simulink model "NMPC_4VEH_4TL"  (R2022b)
settings: Solver=ode4  StartTime=0.0  StopTime=1950  FixedStep=0.1  RelTol=1e-3
PostLoadFcn:
  | , if any(exist('dsrtsu_mdlpostloadfcn', 'file') == [2, 3, 6]), try dsrtsu_mdlpostloadfcn('Execute', bdroot); catch fprintf('Error in PostLoadFcn (dsrtsu_mdlpostloadfcn) for model "%s":\n %s\n', bdroot, lasterr); end, end,
values from neighbouring files (symbols this model uses):
  k_road_map = k_road_map(:)    [NMPC_init_4veh_4TL.m]
  N = 35    [ACADO_4veh_4TL.m]    (also in ACADO_4veh_4TL_BACKUP.m; NMPC_chebyshev_grid.m; NMPC_init_4veh_4TL.m; debug_vincoli_violati.m = 40)
  N_iter = 1    [NMPC_init_4veh_4TL.m]
  N_Jterms = length(Qx1)    [NMPC_init_4veh_4TL.m]
  NMPC_Wmat1 = reshape(W1.',1,[])    [NMPC_init_4veh_4TL.m]
  NMPC_WNmat1 = reshape(WN1.',1,[])    [NMPC_init_4veh_4TL.m]
  t_dwell = 7    [ACADO_4veh_4TL.m]    (also in ACADO_4veh_4TL_BACKUP.m; NMPC_init_4veh_4TL.m)
  t_offset = 0    [NMPC_init_4veh_4TL.m]
  time_bag_sim = (0:1:round(time_bag(end))-1)'    [NMPC_init_4veh_4TL.m]
  time_grid = T_hor*tau_grid    [NMPC_init_4veh_4TL.m]
  tl_state_sim = zeros(round(time_bag(end))-1,size(tl_col,2))    [NMPC_init_4veh_4TL.m]
  Ts = Ts_ctrl    (= 1)    [NMPC_init_4veh_4TL.m]
  Vmax = 50    [NMPC_init_4veh_4TL.m]
  xInit = [0 0 0 -9 0 0 -19 0 0 -29 0 0]    [NMPC_init_4veh_4TL.m]
undefined symbols (not defined in the file or in its folder): ds, s_start
libraries: simulink x1
(part 1 of 2)
settings Model: DSRTSU_INTERNAL_RTI_VER=450  DSRTSU_INTERNAL_RTI_TYPE=rti1401  DSRTSU_INTERNAL_RTIFPGA=40  Creator=d068515  LastModifiedBy=ricca
settings DataIOCC: SaveFormat=StructureWithTime
settings OptimizationCC: BlockReduction=off  LifeSpan=inf
settings DebuggingCC: SFExecutionAtInitializationDiag=none  SFMachineParentedDataDiag=warning  ArithmeticOperatorsInVariantConditions=warning
settings HardwareCC: ProdBitPerSizeT=32  ProdBitPerPtrDiffT=32  ProdEndianess=BigEndian  ProdWordSize=32  ProdHWDeviceType=Generic->Custom  TargetIntDivRoundTo=Zero  TargetEndianess=BigEndian  TargetHWDeviceType=Generic->Custom
settings SFSimCC: CustomCodeUndefinedFunction=UseInterfaceOnly
settings RTWCC: Description=dSPACE DS1401 Hardware Platform  SystemTargetFile=rti1401.tlc  MakeCommand=make_rti  TemplateMakefile=rti1401.tmf
settings CodeAppCC: StateflowObjectComments=on
settings STFCustomTargetCC: ParMdlRefBuildCompliant=on  GRTInterface=on  SystemTargetFile=rti1401.tlc
settings GRTTargetCC: TargetLangStandard=C89/C90 (ANSI)  CompOptLevelCompliant=off  ConcurrentExecutionCompliant=off  CombineOutputUpdateFcns=off  MatFileLogging=off  CPPClassGenCompliant=off  GRTInterface=on  UseToolchainInfoCompliant=off  ExtModeMexFile=noextcomm

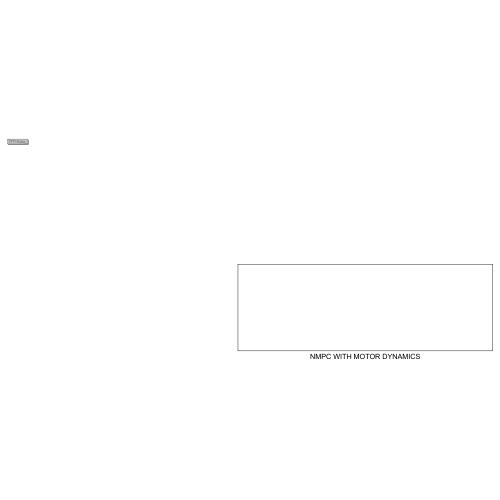
[thumbnail: Simulink's stored preview of the top-level diagram]
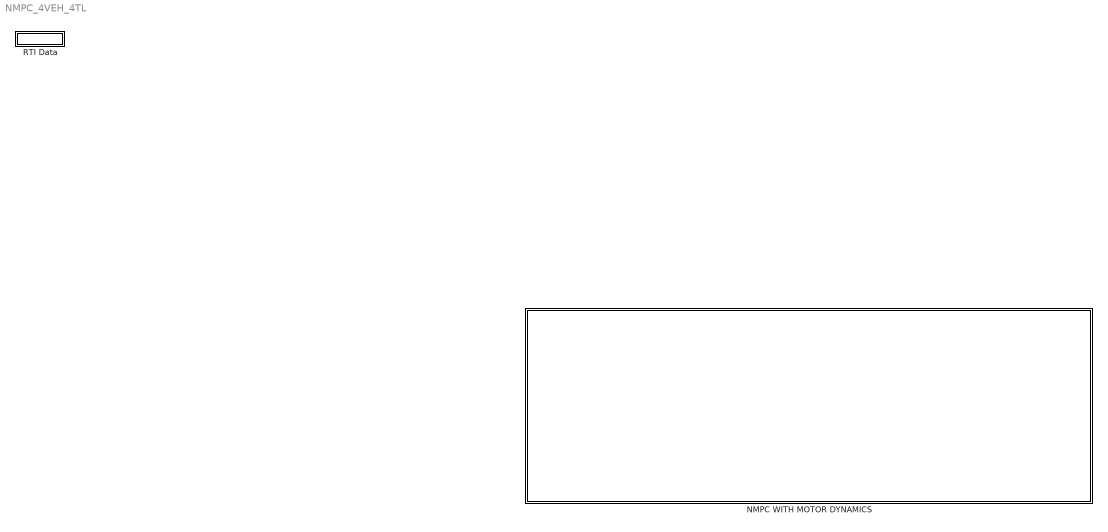
== system NMPC_4VEH_4TL ==
  NMPC WITH MOTOR DYNAMICS : Subsystem
  RTI Data : Subsystem  Tag=struct('RTIDataServer',struct('RTIDataServerVs','2','RTIModelDescription','struct(''main'',''TC_RAF_2014b'',''sub'','''',''isMp'',0)'))  LoadFcn="if exist('rtidc'), try,  rtidc('DataHostBlockClbLoad', gcbh); catch, disp(['Warning: ''LoadFcn'' for RTI Data block failed: ' lasterr]); end, end,"  mask(RTI_DATA_HOST){}
      mask help:
      | RTI Data Block.
      | This block is used by RTI to store internal model-dependent data.
      | Please keep this block on the root level of the model. Deleting this block will result in data loss.
      |
      | NEVER DELETE OR COPY THIS BLOCK!
      settings: CopyFcn="if exist('rtidc'), try,  rtidc('DataHostBlockClbCopy', gcbh); catch, disp(['Warning: ''CopyFcn'' for RTI Data block failed: ' lasterr]); end, end,"  DeleteFcn="if exist('rtidc'), try,  rtidc('DataHostBlockClbDelete', gcbh); catch, disp(['Warning: ''DeleteFcn'' for RTI Data block failed: ' lasterr]); end, end,"  ModelCloseFcn="if exist('rtidc'), try,  rtidc('DataHostBlockClbModelClose', gcbh); catch, disp(['Warning: ''ModelCloseFcn'' for RTI Data block failed: ' lasterr]); end, end,"  PreSaveFcn="if exist('rtidc'), try,  rtidc('DataHostBlockClbPreSave', gcbh); catch, disp(['Warning: ''PreSaveFcn'' for RTI Data block failed: ' lasterr]); end, end,"  PostSaveFcn="if exist('rtidc'), try,  rtidc('DataHostBlockClbPostSave', gcbh); catch, disp(['Warning: ''PostSaveFcn'' for RTI Data block failed: ' lasterr]); end, end,"  NameChangeFcn="if exist('rtidc'), try,  rtidc('DataHostBlockClbNameChange', gcbh); catch, disp(['Warning: ''NameChangeFcn'' for RTI Data block failed: ' lasterr]); end, end,"
      mask Help:
      | RTI Data Block.
      | This block is used by RTI to store internal model-dependent data.
      | Please keep this block on the root level of the model. Deleting this block will result in data loss.
      | 
      | NEVER DELETE OR COPY THIS BLOCK!
      mask Display:
      | text(0.5, 0.5, 'RTI Data', 'HorizontalAlignment', 'center');
      | plot([1 0]);

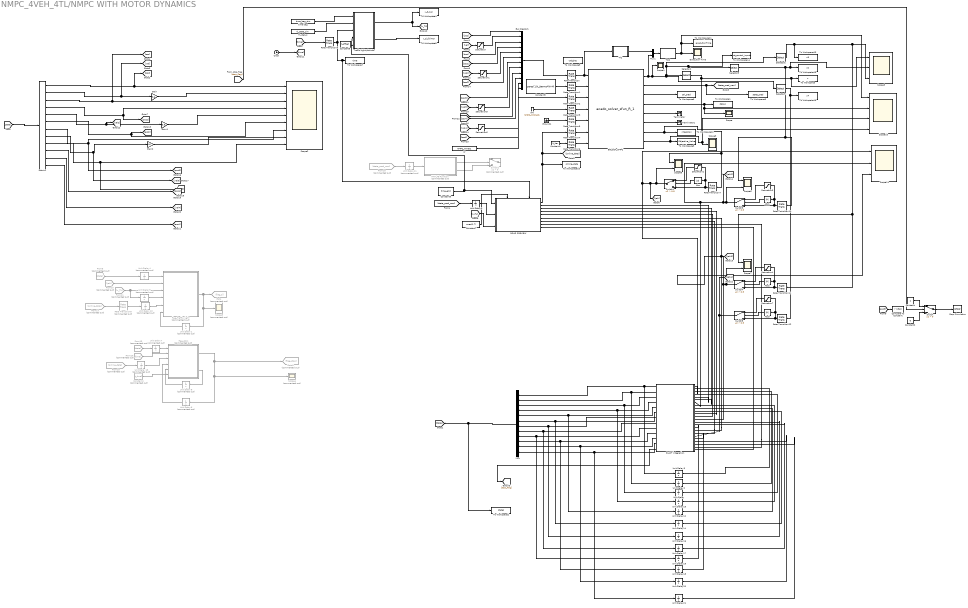
== system NMPC_4VEH_4TL/NMPC WITH MOTOR DYNAMICS ==
  Abs{,1..3} (4 alike) : Abs  SaturateOnIntegerOverflow=off
  BGLOSA_NMPC : S-Function  FunctionName=acado_solver_sfun_R_1  Parameters=xInit, zInit, uInit, NMPC_Wmat1, NMPC_WNmat1, bValues  SFunctionDeploymentMode=off  EnableBusSupport=off  mask(Legacy Function){SFunctionSpec=acado_step(ACADOinput u1[1], ACADOoutput y1[1]), ShowSpec=on}
      mask prompts: ShowSpec "Display function specification"
      mask help:
      | This block allows you to call the legacy functions specified by the following Legacy Code Tool definition:
      | def.SFunctionName = 'acado_solver_sfun';
      | def.OutputFcnSpec = 'acado_step(ACADOinput u1[1], ACADOoutput y1[1])';
      | def.StartFcnSpec = 'acado_initialize( void )';
      | def.TerminateFcnSpec = 'acado_cleanup( void )';
      | def.HeaderFiles = {'acado_common.h', 'acado_solver_sfunction.h'};
      | def.SourceFiles = {'acado_solver.c', 'acado_integrator.c', 'acado_auxiliary_functions.c', 'acado_solver_sfunction.c', 'acado_qpoases_interface.cpp', 'qpoases/SRC/Bounds.cpp', 'qpoases/SRC/Constraints.cpp', 'qpoases/SRC/CyclingManager.cpp', 'qpoases/SRC/Indexlist.cpp', 'qpoases/SRC/MessageHandling.cpp', 'qpoases/SRC/QProblem.cpp', 'qpoases/SRC/QProblemB.cpp', 'qpoases/SRC/SubjectTo.cpp', 'qpoases/SRC/Utils.cpp', 'qpoases/SRC/EXTRAS/SolutionAnalysis.cpp'};
      | def.IncPaths = {'qpoases', 'qpoases/INCLUDE', 'qpoases/SRC'};
      | def.Options.language = 'C++';
      mask Help: <p>This block was generated automatically by the Legacy Code Tool. For detailed help on this tool, call<a href="matlab:legacy_code('help')"> legacy_code('help')</a>.</p>
      mask Callback ShowSpec:
      | if strcmp(get_param(gcbh, 'ShowSpec'), 'on')
      |   set_param(gcbh, 'MaskDisplay', sprintf('fprintf(''%s'');', get_param(gcbh, 'SFunctionSpec')));
      | else
      |   set_param(gcbh, 'MaskDisplay', sprintf('fprintf(''%s'');', get_param(gcbh, 'FunctionName')));
      | end
      mask Display: fprintf('acado_step(ACADOinput u1[1], ACADOoutput y1[1])');
  Bus Creator1 : BusCreator  Inputs=12
  Clock : Clock
  Compare To Constant : simulink/Logic and Bit Operations/Compare To Constant  relop=>  const=1940  OutDataTypeStr=boolean
  Constant : Constant
  Constant1 : Constant  Value=N_iter
  Constant2 : Constant  Value=0
  Constant3 : Constant  Value=time_grid
  Constant4 : Constant  Commented=on  Value=t_dwell
  Constant5 : Constant  Value=zeros(1,N_Jterms*N+4)
  Constant6 : Constant  Value=t_offset
  Constant7 : Constant  Value=ones(1,7)
  Demux : Demux  Outputs=12
  Execution Time : Scope
  From10 : From  Commented=on  GotoTag=jerk
  From11 : From  Commented=on  GotoTag=x_TL
  From13 : From  Commented=on  GotoTag=state
  From17 : From  Commented=on  GotoTag=online_data
  From18 : From  Commented=on  GotoTag=state_pred_new
  From19 : From  Commented=on  GotoTag=online_data
  From20 : From  Commented=on  GotoTag=time
  From5 : From  Commented=on  GotoTag=state
  Gain : Gain  Gain=3.6
  Gain1 : Gain  Gain=3.6
  Gain2 : Gain  Gain=3.6
  Goto : Goto  Commented=on  GotoTag=flag_tl
  Goto8 : Goto  Commented=on  GotoTag=flag_stop
  Ground1 : Ground
  MATLAB Function : MATLAB Function  Commented=on  TreatAsAtomicUnit=on
  Mux : Mux  Inputs=12
  Mux1 : Mux  Inputs=2
  PLANT integration : MATLAB Function  TreatAsAtomicUnit=on
  ROAD PREVIEW : Subsystem
      settings: PortSchema="{\"entries\":[{\"content\":{\"sides\":[{\"content\":{\"connectorIds\":[\"In1\",\"In2\",\"In3\"]},\"type\":\"ConnectorPlacement.EquallySpacedRectSide\",\"uuid\":\"89746bc5-bd2f-4e61-9556-28242176c46a\"},{\"content\":{\"connectorIds\":[\"Out1\",\"Out2\",\"Out3\",\"Out4\",\"Out5\",\"Out6\",\"Out7\",\"Out8\",\"Out9\"],\"side\":\"RIGHT\"},\"type\":\"ConnectorPlacement.EquallySpacedRectSide\",\"uuid\":\"fa5eae8e-eb55-42b4-8d8b-02c8b36cc91d\"},{\"content\":{\"connectorIds\":[\"In4\",\"In5\"],\"side\":\"TOP\"},\"type\":\"ConnectorPlacement.EquallySpacedRectSide\",\"uuid\":\"5942e98b-dfb5-4e56-acd3-edfb2315bb7f\"}]},\"type\":\"ConnectorPlacement.EquallySpacedConnector\",\"uuid\":\"ba8f73d0-227f-4198-ac0b-e11b2a073141\"}],\"packageUris\":[\"http://schema.mathworks.com/mf0/Connector/R2020b\"],\"version\":\"1.0\"}"
  Rate Transition : RateTransition  Deterministic=off  InitialCondition=xInit  OutPortSampleTime=Ts
  Rate Transition{1..6} (6 alike) : RateTransition  Deterministic=off  OutPortSampleTime=Ts
  Rate Transition{7,10..12} (4 alike) : RateTransition  Deterministic=off  OutPortSampleTime=0.1
  Rate Transition8 : RateTransition  Commented=on  InitialCondition=zeros(1665,1)  OutPortSampleTime=Ts
  Rate Transition9 : RateTransition  OutPortSampleTime=Ts
  Saturation{,1,5..6} (4 alike) : Saturate  UpperLimit=50/3.6  LowerLimit=0
  Saturation{2..4,7} (4 alike) : Saturate  UpperLimit=0.1  LowerLimit=-0.1
  Scope : Scope
  Scope1 : Scope
  Scope10 : Scope  NumInputPorts=4
  Scope11 : Scope  NumInputPorts=3
  Scope2 : Scope  NumInputPorts=9
  Scope3 : Scope
  Scope4 : Scope  Commented=on
  Scope5 : Scope  Commented=on
  Scope6 : Scope  NumInputPorts=2
  Scope7 : Scope  NumInputPorts=2
  Scope8 : Scope  NumInputPorts=2
  Scope9 : Scope  NumInputPorts=3
  Selector1 : Selector  NumberOfDimensions=2  InputPortWidth=3  IndexOptions=Index vector (dialog),Index vector (dialog)  Indices=[1],1  OutputSizes=1,1
  Selector2 : Selector  NumberOfDimensions=2  InputPortWidth=3  IndexOptions=Index vector (dialog),Index vector (dialog)  Indices=[1],3  OutputSizes=1,1
  Selector3 : Selector  NumberOfDimensions=2  InputPortWidth=3  IndexOptions=Index vector (dialog),Index vector (dialog)  Indices=[1],2  OutputSizes=1,1
  Selector5 : Selector  NumberOfDimensions=2  InputPortWidth=3  IndexOptions=Index vector (dialog),Index vector (dialog)  Indices=[1],4  OutputSizes=1,1
  Stop Simulation : Stop
  Switch : Switch  Criteria=u2 > Threshold  SaturateOnIntegerOverflow=off  InputSameDT=off
  Switch{1,3..5} (4 alike) : Switch  Criteria=u2 > Threshold  Threshold=0.5  SaturateOnIntegerOverflow=off  InputSameDT=off
  Switch2 : Switch  Commented=on  Criteria=u2 > Threshold  SaturateOnIntegerOverflow=off  InputSameDT=off
  TIC : MATLAB Function  TreatAsAtomicUnit=on
  TL status : Constant  Value=tl_state_sim  OutDataTypeStr=double
  TOC : MATLAB Function  TreatAsAtomicUnit=on
  Terminator : Terminator
  Terminator1 : Terminator
  To Workspace : ToWorkspace  VariableName=u  SaveFormat=Structure With Time  SampleTime=-1
  To Workspace1 : ToWorkspace  VariableName=status  SaveFormat=Structure With Time  SampleTime=-1
  To Workspace10 : ToWorkspace  VariableName=online_data  SaveFormat=Structure With Time  SampleTime=-1
  To Workspace11 : ToWorkspace  VariableName=executionTime  SaveFormat=Structure With Time  SampleTime=-1
  To Workspace12 : ToWorkspace  VariableName=nIteration  SaveFormat=Structure With Time  SampleTime=-1
  To Workspace13 : ToWorkspace  VariableName=u3  SaveFormat=Structure With Time  SampleTime=-1
  To Workspace14 : ToWorkspace  VariableName=first_control_inputs  SaveFormat=Timeseries  SampleTime=-1
  To Workspace15 : ToWorkspace  VariableName=u2  SaveFormat=Structure With Time  SampleTime=-1
  To Workspace16 : ToWorkspace  VariableName=u4  SaveFormat=Structure With Time  SampleTime=-1
  To Workspace2 : ToWorkspace  VariableName=states  SaveFormat=Structure With Time  SampleTime=-1
  To Workspace3 : ToWorkspace  VariableName=Objective_Value  SaveFormat=Structure With Time  SampleTime=-1
  To Workspace4 : ToWorkspace  VariableName=x_tl_hor  SaveFormat=Structure With Time  SampleTime=-1
  To Workspace5 : ToWorkspace  VariableName=state_pred  SaveFormat=Structure With Time  SampleTime=-1
  To Workspace6 : ToWorkspace  VariableName=ctrl_pred  SaveFormat=Structure With Time  SampleTime=-1
  To Workspace7 : ToWorkspace  VariableName=time  SaveFormat=Structure With Time  SampleTime=-1
  To Workspace8 : ToWorkspace  VariableName=x_tl_fullHor  SaveFormat=Structure With Time  SampleTime=-1
  To Workspace9 : ToWorkspace  VariableName=weights  SaveFormat=Structure With Time  SampleTime=-1
  Traffic Light planner : MATLAB Function  TreatAsAtomicUnit=on
  Unit Delay : UnitDelay  InitialCondition=xInit(3)  SampleTime=-1  HasFrameUpgradeWarning=on
  Unit Delay1 : UnitDelay  Commented=on  InitialCondition=zeros(1,11)  SampleTime=-1  HasFrameUpgradeWarning=on
  Unit Delay10 : UnitDelay  Commented=on  InitialCondition=zeros(50*(N+1),1)  SampleTime=-1  HasFrameUpgradeWarning=on
  Unit Delay11 : UnitDelay  Commented=on  InitialCondition=xInit.*ones(N+1,9)  SampleTime=-1  HasFrameUpgradeWarning=on
  Unit Delay12 : UnitDelay  InitialCondition=xInit(5)  SampleTime=-1  HasFrameUpgradeWarning=on
  Unit Delay13 : UnitDelay  Commented=on  InitialCondition=zeros(50*(N+1),1)  SampleTime=-1  HasFrameUpgradeWarning=on
  Unit Delay14 : UnitDelay  InitialCondition=xInit(6)  SampleTime=-1  HasFrameUpgradeWarning=on
  Unit Delay15 : UnitDelay  InitialCondition=xInit(4)  SampleTime=-1  HasFrameUpgradeWarning=on
  Unit Delay16 : UnitDelay  InitialCondition=xInit(7)  SampleTime=-1  HasFrameUpgradeWarning=on
  Unit Delay17 : UnitDelay  InitialCondition=xInit(8)  SampleTime=-1  HasFrameUpgradeWarning=on
  Unit Delay18 : UnitDelay  InitialCondition=xInit(10)  SampleTime=-1  HasFrameUpgradeWarning=on
  Unit Delay19 : UnitDelay  InitialCondition=xInit(9)  SampleTime=-1  HasFrameUpgradeWarning=on
  Unit Delay2 : UnitDelay  InitialCondition=xInit(2)  SampleTime=-1  HasFrameUpgradeWarning=on
  Unit Delay20 : UnitDelay  InitialCondition=xInit(11)  SampleTime=-1  HasFrameUpgradeWarning=on
  Unit Delay21 : UnitDelay  InitialCondition=xInit(12)  SampleTime=-1  HasFrameUpgradeWarning=on
  Unit Delay3 : UnitDelay  InitialCondition=xInit(1)  SampleTime=-1  HasFrameUpgradeWarning=on
  Unit Delay4 : UnitDelay  Commented=on  InitialCondition=xInit  SampleTime=-1  HasFrameUpgradeWarning=on
  Unit Delay5 : UnitDelay  Commented=on  InitialCondition=zeros(N+1,12)  SampleTime=-1  HasFrameUpgradeWarning=on
  Unit Delay6 : UnitDelay  Commented=on  InitialCondition=zeros(1,7)  SampleTime=-1  HasFrameUpgradeWarning=on
  Unit Delay7 : UnitDelay  Commented=on  InitialCondition=xInit  SampleTime=-1  HasFrameUpgradeWarning=on
  Unit Delay8 : UnitDelay  Commented=on  InitialCondition=zeros(1,7)  SampleTime=-1  HasFrameUpgradeWarning=on
  Unit Delay9 : UnitDelay  InitialCondition=xInit.*ones(N+1,12)  SampleTime=-1  HasFrameUpgradeWarning=on
  W : Constant  Value=NMPC_Wmat1  OutDataTypeStr=double
  "WN " : Constant  Value=NMPC_WNmat1  OutDataTypeStr=double
  flag_Stop : MATLAB Function  Commented=on  TreatAsAtomicUnit=on
  flag_Traffic_Light : MATLAB Function  Commented=on  TreatAsAtomicUnit=on
  time bag : Constant  Value=time_bag_sim  OutDataTypeStr=double
  wires:
  BGLOSA_NMPC/3 -> To Workspace6/1  "Control Inputs Prediction"
  BGLOSA_NMPC/4 -> To Workspace1/1, Scope/1, Scope10/2  "Status QP Solver"
  Constant1/1 -> Rate Transition6/1  "Number of iterations"
  BGLOSA_NMPC/8 -> Scope10/3, Scope3/1, To Workspace3/1  "NMPC Objective Value"
  Bus Creator1/1 -> Rate Transition/1  "States"
  BGLOSA_NMPC/1 -> Selector5/1, Selector2/1, Selector3/1, To Workspace14/1, Selector1/1, Scope1/1, Mux1/2  "First Control Input"
  BGLOSA_NMPC/5 -> Terminator/1  "KKT optimization tolerance"
  BGLOSA_NMPC/6 -> Terminator1/1  "(no timing)"
  Ground1/1 -> Rate Transition5/1  "Constraints"
  BGLOSA_NMPC/7 -> Scope10/4, To Workspace12/1
  Rate Transition1/1 -> BGLOSA_NMPC/2
  Rate Transition2/1 -> BGLOSA_NMPC/3
  Rate Transition6/1 -> BGLOSA_NMPC/7
  Rate Transition3/1 -> BGLOSA_NMPC/4
  Rate Transition5/1 -> BGLOSA_NMPC/5
  Rate Transition4/1 -> BGLOSA_NMPC/6
  BGLOSA_NMPC/2 -> To Workspace5/1, [state_pred_new]  "States prediction"
  Constant5/1 -> Rate Transition1/1
  Demux/1 -> [pos], Scope2/1
  Demux/2 -> Gain/1, [vel]
  Demux/3 -> [acc], Scope2/3
  Unit Delay3/1 -> PLANT integration/2(s0)
  ROAD PREVIEW/1(Online Data) -> Rate Transition4/1, [online_data], To Workspace10/1  "Online Data"
  "WN "/1 -> Rate Transition3/1  "Terminal Cost Matrix"
  Selector1/1 -> Rate Transition7/1, Scope8/1, Scope9/1, To Workspace/1
  Unit Delay/1 -> PLANT integration/4(a0)
  Unit Delay2/1 -> PLANT integration/3(v0)
  Mux/1 -> [state], To Workspace2/1
  [state] -> Demux/1
  [pos] -> Bus Creator1/1
  [vel] -> Saturation/1
  [acc] -> Bus Creator1/3
  [state_pred_new] -> Unit Delay9/1
  From5/1 -> Unit Delay4/1
  From10/1 -> flag_Traffic_Light/2(jerk)
  [x_TL] -> ROAD PREVIEW/3(x_TL)
  From11/1 -> flag_Traffic_Light/3(x_TL), Unit Delay5/1
  flag_Traffic_Light/1(flag_mpc) -> Unit Delay1/1, Scope5/1, Goto/1
  Unit Delay1/1 -> flag_Traffic_Light/6(flag_old)
  Unit Delay4/1 -> flag_Traffic_Light/1(state)
  Unit Delay5/1 -> flag_Traffic_Light/4(x_TL_old)
  Unit Delay7/1 -> flag_Stop/1(state)
  Unit Delay6/1 -> flag_Stop/4(flag_old)
  flag_Stop/1(flag_mpc) -> Goto8/1, Unit Delay6/1, Scope4/1
  From20/1 -> flag_Stop/2(time)
  From13/1 -> Unit Delay7/1
  Constant7/1 -> ROAD PREVIEW/4(x_stop)
  Unit Delay9/1 -> ROAD PREVIEW/2(state_pred_old)
  time bag/1 -> Traffic Light planner/1(time_bag)
  TL status/1 -> Traffic Light planner/2(tl_col)
  Rate Transition9/1 -> ROAD PREVIEW/5(time_cur), To Workspace7/1, Traffic Light planner/3(time)
  From17/1 -> Rate Transition8/1
  Unit Delay10/1 -> flag_Traffic_Light/5(online_data)
  flag_Stop/2(time_flag) -> Unit Delay8/1
  Unit Delay8/1 -> flag_Stop/5(time_flag_memory)
  Saturation/1 -> Bus Creator1/2
  [pos3] -> Compare To Constant/1
  Constant/1 -> Switch/1
  Constant2/1 -> Switch/3
  Switch/1 -> Stop Simulation/1
  Rate Transition8/1 -> Unit Delay10/1
  From19/1 -> Unit Delay13/1
  Unit Delay13/1 -> flag_Stop/3(online_data)
  Switch1/1 -> PLANT integration/1(u), Scope11/1, [jerk], Scope8/2
  Rate Transition7/1 -> Saturation2/1, Abs/1, Switch1/3
  Abs/1 -> Switch1/2
  Saturation2/1 -> Switch1/1
  Gain/1 -> Scope2/2
  Constant4/1 -> flag_Stop/6(t_dwell)
  [time] -> Rate Transition9/1
  Constant6/1 -> Traffic Light planner/4(t_offset)
  Rate Transition/1 -> TIC/1(u), BGLOSA_NMPC/1
  Mux1/1 -> TOC/1(u)
  TIC/1(y) -> Mux1/1
  W/1 -> Rate Transition2/1  "Stage Cost Matrix"
  From18/1 -> Unit Delay11/1
  Unit Delay11/1 -> MATLAB Function/1(state_pred)
  MATLAB Function/1(flag) -> Switch2/2
  MATLAB Function/2(NMPC_Wmat1) -> Switch2/3
  Traffic Light planner/1(x_TL) -> To Workspace4/1, [x_TL]
  Traffic Light planner/2(data) -> To Workspace8/1
  Clock/1 -> [time]
  ROAD PREVIEW/2(Outport) -> PLANT integration/5(red_stopline_hold)
  ROAD PREVIEW/3(Outport1) -> PLANT integration/6(s_hold)
  Demux/4 -> [pos2], Scope2/4
  Demux/5 -> Gain1/1, [vel2]
  Demux/6 -> [acc2], Scope2/6
  Gain1/1 -> Scope2/5
  Saturation1/1 -> Bus Creator1/5
  [vel2] -> Saturation1/1
  [pos2] -> Bus Creator1/4
  [acc2] -> Bus Creator1/6
  Selector3/1 -> Rate Transition10/1, Scope6/1, Scope9/2, To Workspace15/1
  Rate Transition10/1 -> Saturation3/1, Abs1/1, Switch3/3
  Saturation3/1 -> Switch3/1
  Abs1/1 -> Switch3/2
  Unit Delay15/1 -> PLANT integration/8(s02)
  Unit Delay12/1 -> PLANT integration/9(v02)
  Unit Delay14/1 -> PLANT integration/10(a02)
  ROAD PREVIEW/4(Outport2) -> PLANT integration/11(red_stopline_hold2)
  ROAD PREVIEW/5(Outport3) -> PLANT integration/12(s_hold2)
  Selector2/1 -> Scope9/3, Scope7/1, Rate Transition11/1, To Workspace13/1
  Rate Transition11/1 -> Saturation4/1, Abs2/1, Switch4/3
  Saturation4/1 -> Switch4/1
  Abs2/1 -> Switch4/2
  Switch4/1 -> Scope11/3, [jerk3], PLANT integration/13(u3), Scope7/2
  Unit Delay16/1 -> PLANT integration/14(s03)
  Unit Delay17/1 -> PLANT integration/15(v03)
  ROAD PREVIEW/6(Outport4) -> PLANT integration/17(red_stopline_hold3)
  ROAD PREVIEW/7(Outport5) -> PLANT integration/18(s_hold3)
  Demux/7 -> Scope2/7, [pos3]
  Demux/8 -> [vel3], Gain2/1
  Gain2/1 -> Scope2/8
  Demux/9 -> Scope2/9, [acc3]
  TOC/1(y) -> Scope10/1, To Workspace11/1, Execution Time/1
  [pos3] -> Bus Creator1/7
  [acc3] -> Bus Creator1/9
  [vel3] -> Saturation5/1
  Saturation5/1 -> Bus Creator1/8
  [stop_flag] -> Switch/2
  Switch3/1 -> Scope11/2, PLANT integration/7(u2), [jerk2], Scope6/2
  Constant3/1 -> ROAD PREVIEW/1(time_grid), Traffic Light planner/5(time_grid)
  ROAD PREVIEW/8(Outport6) -> PLANT integration/23(red_stopline_hold4)
  ROAD PREVIEW/9(Outport7) -> PLANT integration/24(s_hold4)
  Unit Delay20/1 -> PLANT integration/21(v04)
  Unit Delay21/1 -> PLANT integration/22(a04)
  Demux/10 -> [pos4]
  Demux/11 -> [vel4]
  Demux/12 -> [acc4]
  [vel4] -> Saturation6/1
  [pos4] -> Bus Creator1/10
  Saturation6/1 -> Bus Creator1/11
  [acc4] -> Bus Creator1/12
  Selector5/1 -> Rate Transition12/1, To Workspace16/1
  Rate Transition12/1 -> Saturation7/1, Abs3/1, Switch5/3
  Saturation7/1 -> Switch5/1
  Abs3/1 -> Switch5/2
  Switch5/1 -> [jerk4], PLANT integration/19(u4)
  PLANT integration/1(s) -> Unit Delay3/1, Mux/1
  PLANT integration/2(v) -> Unit Delay2/1, Mux/2
  PLANT integration/3(a) -> Unit Delay/1, Mux/3
  PLANT integration/4(s2) -> Unit Delay15/1, Mux/4
  PLANT integration/5(v2) -> Unit Delay12/1, Mux/5
  PLANT integration/6(a2) -> Unit Delay14/1, Mux/6
  PLANT integration/7(s3) -> Unit Delay16/1, Mux/7
  PLANT integration/8(v3) -> Unit Delay17/1, Mux/8
  PLANT integration/9(a3) -> Unit Delay19/1, Mux/9
  PLANT integration/10(s4) -> Unit Delay18/1, Mux/10
  PLANT integration/11(v4) -> Unit Delay20/1, Mux/11
  PLANT integration/12(a4) -> Unit Delay21/1, Mux/12
  Unit Delay19/1 -> PLANT integration/16(a03)
  Unit Delay18/1 -> PLANT integration/20(s04)
  PLANT integration/13(stop_flag) -> [stop_flag]

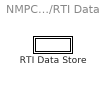
== system NMPC_4VEH_4TL/RTI Data ==
  RTI Data Store : Subsystem  Tag="struct('private',struct('version',struct('dsVer',uint32(2),'dsVerCreation',uint32(2),'RTI',struct('ver','7.3','type','RTI1401')),'access',struct('type','Model','isPerm',1,'created',['23-Jan-2024 14:08:40'],'modified',['23-Jan-2024 15:26:34'],'location','')),'public',struct('main',struct('data',[]),'sub',struct('name',{{'TC_RAF_2014b'}},'data',{{struct('TH',struct('thTaskInfo',struct('taskType',{'TIMER','HWINT','TMRINT','SWINT','GLINT'},'tasksNumOf',{1,0,0,0,0},'srcIds',{{'TIMERA'},{},{},{},{}},'taskNames',{{['Timer Task 1']},{},{},{},{}})),'th_tc',struct('dataType','TASK','taskGroupId','','taskGroupList',{{}},'taskSchedulingPolicy','FCFS','taskType','TIMER','blkh',-1,'srcId','TIMERA','srcSgnName',['Timer A interrupt'],'srcCpuName','','taskName',['Timer Task 1  [0.01] s'],'taskNameDisplayExt','','smplTime',0.01,'smplTimeOffs',0,'hasFixedPriority',0,'priority',1,'hasFixedOvc',0,'ovcType',1,'ovcMax',1),'tc_th',struct('dataType','TASK','taskGroupId','','taskGroupList',{{}},'taskSchedulingPolicy','FCFS','taskType','TIMER','blkh',-1,'srcId','TIMERA','srcSgnName',['Timer A interrupt'],'srcCpuName','','taskName',['Timer Task 1  [0.01] s'],'taskNameDisplayExt','','smplTime',0.01,'smplTimeOffs',0,'hasFixedPriority',0,'priority',1,'hasFixedOvc',0,'ovcType',1,'ovcMax',1))}})))"  mask(RTI_DATA_STORE){}
      mask help:
      | RTI Data Store Block. This block is used by RTI to store internal model dependent data. Deleting this block will result in data loss.
      |
      | NEVER DELETE, COPY, OR MODIFY THIS BLOCK!
      mask Help:
      | RTI Data Store Block. This block is used by RTI to store internal model dependent data. Deleting this block will result in data loss.
      | 
      | NEVER DELETE, COPY, OR MODIFY THIS BLOCK!
      mask Display: text(0.5, 0.5, ' ', 'HorizontalAlignment', 'center');

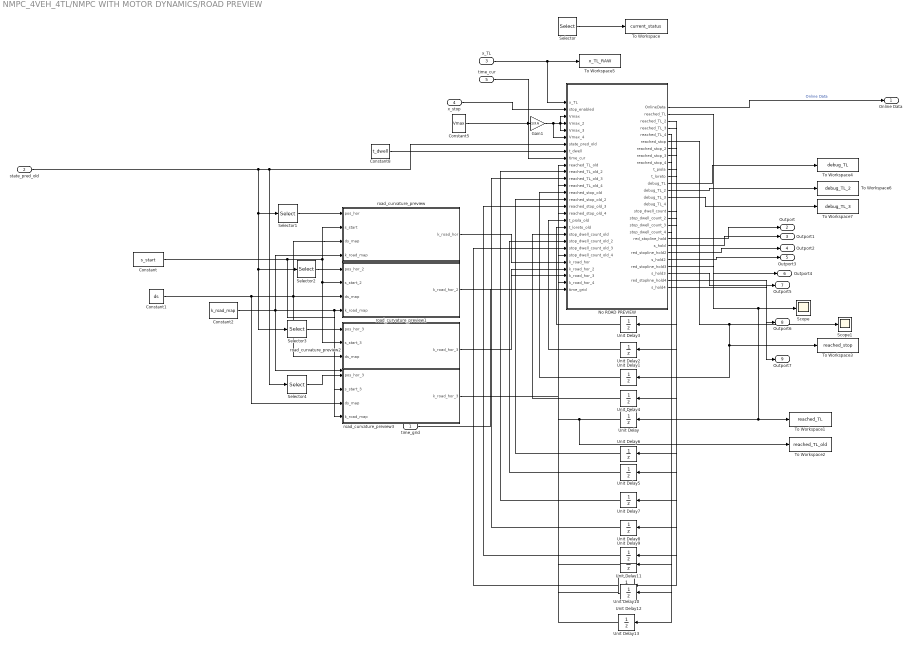
== system NMPC_4VEH_4TL/NMPC WITH MOTOR DYNAMICS/ROAD PREVIEW ==
  time_grid : Inport
  state_pred_old : Inport  Port=2
  x_TL : Inport  Port=3
  x_stop : Inport  Port=4
  time_cur : Inport  Port=5
  Constant : Constant  Value=s_start
  Constant1 : Constant  Value=ds
  Constant2 : Constant  Value=k_road_map
  Constant5 : Constant  Value=Vmax
  Constant8 : Constant  Value=t_dwell  VectorParams1D=off
  Gain1 : Gain  Gain=1/3.6
  No ROAD PREVIEW : MATLAB Function  TreatAsAtomicUnit=on  SystemSampleTime=Ts
  Scope : Scope
  Scope1 : Scope
  Selector : Selector  NumberOfDimensions=2  InputPortWidth=3  IndexOptions=Index vector (dialog),Select all  Indices=1,1  OutputSizes=1,1
  Selector1 : Selector  NumberOfDimensions=2  InputPortWidth=3  IndexOptions=Select all,Index vector (dialog)  Indices=[1 3],1  OutputSizes=1,1
  Selector2 : Selector  NumberOfDimensions=2  InputPortWidth=3  IndexOptions=Select all,Index vector (dialog)  Indices=[1 3],4  OutputSizes=1,1
  Selector3 : Selector  NumberOfDimensions=2  InputPortWidth=3  IndexOptions=Select all,Index vector (dialog)  Indices=[1 3],7  OutputSizes=1,1
  Selector4 : Selector  NumberOfDimensions=2  InputPortWidth=3  IndexOptions=Select all,Index vector (dialog)  Indices=[1 3],10  OutputSizes=1,1
  To Workspace : ToWorkspace  VariableName=current_status  SaveFormat=Structure With Time  SampleTime=-1
  To Workspace1 : ToWorkspace  VariableName=reached_TL  SaveFormat=Structure With Time  SampleTime=-1
  To Workspace2 : ToWorkspace  VariableName=reached_TL_old  SaveFormat=Structure With Time  SampleTime=-1
  To Workspace3 : ToWorkspace  VariableName=reached_stop  SaveFormat=Structure With Time  SampleTime=-1
  To Workspace4 : ToWorkspace  VariableName=debug_TL  SaveFormat=Timeseries  SampleTime=-1
  To Workspace5 : ToWorkspace  VariableName=x_TL_RAW  SaveFormat=Timeseries  SampleTime=-1
  To Workspace6 : ToWorkspace  VariableName=debug_TL_2  SaveFormat=Timeseries  SampleTime=-1
  To Workspace7 : ToWorkspace  VariableName=debug_TL_3  SaveFormat=Timeseries  SampleTime=-1
  Unit Delay{,7..8,11} (4 alike) : UnitDelay  InitialCondition=zeros(1,30)  SampleTime=-1  HasFrameUpgradeWarning=on
  Unit Delay{1,4..6,9..10,12..13} (8 alike) : UnitDelay  InitialCondition=zeros(1,7)  SampleTime=-1  HasFrameUpgradeWarning=on
  Unit Delay2 : UnitDelay  SampleTime=-1  HasFrameUpgradeWarning=on
  Unit Delay3 : UnitDelay  SampleTime=-1  HasFrameUpgradeWarning=on
  road_curvature_preview : MATLAB Function  TreatAsAtomicUnit=on
  road_curvature_preview1 : MATLAB Function  TreatAsAtomicUnit=on
  road_curvature_preview2 : MATLAB Function  TreatAsAtomicUnit=on
  road_curvature_preview3 : MATLAB Function  TreatAsAtomicUnit=on
  Online Data : Outport
  Outport : Outport  Port=2
  Outport1 : Outport  Port=3
  Outport2 : Outport  Port=4
  Outport3 : Outport  Port=5
  Outport4 : Outport  Port=6
  Outport5 : Outport  Port=7
  Outport6 : Outport  Port=8
  Outport7 : Outport  Port=9
  wires:
  No ROAD PREVIEW/1(OnlineData) -> Online Data/1  "Online Data"
  Constant5/1 -> Gain1/1
  Gain1/1 -> No ROAD PREVIEW/3(Vmax), No ROAD PREVIEW/4(Vmax_2), No ROAD PREVIEW/5(Vmax_3), No ROAD PREVIEW/6(Vmax_4)
  state_pred_old/1 -> Selector4/1, No ROAD PREVIEW/7(state_pred_old), Selector3/1, Selector2/1, Selector1/1
  Selector/1 -> To Workspace/1
  No ROAD PREVIEW/2(reached_TL) -> To Workspace1/1, Unit Delay/1, Scope/1
  Unit Delay/1 -> No ROAD PREVIEW/10(reached_TL_old), To Workspace2/1
  x_TL/1 -> No ROAD PREVIEW/1(x_TL), To Workspace5/1
  x_stop/1 -> No ROAD PREVIEW/2(stop_enabled)
  No ROAD PREVIEW/6(reached_stop) -> To Workspace3/1, Unit Delay1/1, Scope1/1
  Unit Delay1/1 -> No ROAD PREVIEW/14(reached_stop_old)
  Constant8/1 -> No ROAD PREVIEW/8(t_dwell)
  No ROAD PREVIEW/10(t_piola) -> Unit Delay2/1
  No ROAD PREVIEW/11(t_loreto) -> Unit Delay3/1
  Unit Delay2/1 -> No ROAD PREVIEW/18(t_piola_old)
  Unit Delay3/1 -> No ROAD PREVIEW/19(t_loreto_old)
  No ROAD PREVIEW/12(debug_TL) -> To Workspace4/1
  Unit Delay4/1 -> No ROAD PREVIEW/20(stop_dwell_count_old)
  No ROAD PREVIEW/16(stop_dwell_count) -> Unit Delay4/1
  No ROAD PREVIEW/20(red_stopline_hold) -> Outport/1
  No ROAD PREVIEW/21(s_hold) -> Outport1/1
  Constant2/1 -> road_curvature_preview3/4(k_road_map), road_curvature_preview1/4(k_road_map), road_curvature_preview/4(k_road_map), road_curvature_preview2/4(k_road_map)
  Constant1/1 -> road_curvature_preview1/3(ds_map), road_curvature_preview2/3(ds_map), road_curvature_preview/3(ds_map), road_curvature_preview3/3(ds_map)
  Constant/1 -> road_curvature_preview/2(s_start), road_curvature_preview2/2(s_start_3), road_curvature_preview1/2(s_start_2), road_curvature_preview3/2(s_start_3)
  road_curvature_preview/1(k_road_hor) -> No ROAD PREVIEW/24(k_road_hor)
  Selector1/1 -> road_curvature_preview/1(pos_hor)
  time_cur/1 -> No ROAD PREVIEW/9(time_cur)
  No ROAD PREVIEW/22(red_stopline_hold2) -> Outport2/1
  No ROAD PREVIEW/23(s_hold2) -> Outport3/1
  No ROAD PREVIEW/17(stop_dwell_count_2) -> Unit Delay5/1
  Unit Delay5/1 -> No ROAD PREVIEW/21(stop_dwell_count_old_2)
  No ROAD PREVIEW/7(reached_stop_2) -> Unit Delay6/1
  Unit Delay6/1 -> No ROAD PREVIEW/15(reached_stop_old_2)
  No ROAD PREVIEW/3(reached_TL_2) -> Unit Delay7/1
  Unit Delay7/1 -> No ROAD PREVIEW/11(reached_TL_old_2)
  road_curvature_preview1/1(k_road_hor_2) -> No ROAD PREVIEW/25(k_road_hor_2)
  Selector2/1 -> road_curvature_preview1/1(pos_hor_2)
  No ROAD PREVIEW/13(debug_TL_2) -> To Workspace6/1
  Selector3/1 -> road_curvature_preview2/1(pos_hor_3)
  road_curvature_preview2/1(k_road_hor_3) -> No ROAD PREVIEW/26(k_road_hor_3)
  No ROAD PREVIEW/14(debug_TL_3) -> To Workspace7/1
  No ROAD PREVIEW/4(reached_TL_3) -> Unit Delay8/1
  Unit Delay8/1 -> No ROAD PREVIEW/12(reached_TL_old_3)
  No ROAD PREVIEW/8(reached_stop_3) -> Unit Delay9/1
  Unit Delay9/1 -> No ROAD PREVIEW/16(reached_stop_old_3)
  No ROAD PREVIEW/18(stop_dwell_count_3) -> Unit Delay10/1
  Unit Delay10/1 -> No ROAD PREVIEW/22(stop_dwell_count_old_3)
  No ROAD PREVIEW/24(red_stopline_hold3) -> Outport4/1
  No ROAD PREVIEW/25(s_hold3) -> Outport5/1
  time_grid/1 -> No ROAD PREVIEW/28(time_grid)
  Selector4/1 -> road_curvature_preview3/1(pos_hor_3)
  road_curvature_preview3/1(k_road_hor_3) -> No ROAD PREVIEW/27(k_road_hor_4)
  No ROAD PREVIEW/5(reached_TL_4) -> Unit Delay11/1
  Unit Delay11/1 -> No ROAD PREVIEW/13(reached_TL_old_4)
  No ROAD PREVIEW/9(reached_stop_4) -> Unit Delay12/1
  Unit Delay12/1 -> No ROAD PREVIEW/17(reached_stop_old_4)
  No ROAD PREVIEW/19(stop_dwell_count_4) -> Unit Delay13/1
  Unit Delay13/1 -> No ROAD PREVIEW/23(stop_dwell_count_old_4)
  No ROAD PREVIEW/26(red_stopline_hold4) -> Outport6/1
  No ROAD PREVIEW/27(s_hold4) -> Outport7/1

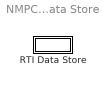
== system NMPC_4VEH_4TL/RTI Data/RTI Data Store ==
  RTI Data Store : Subsystem  mask(RTI_DATA_STORE){}
      mask help:
      | RTI Data Store Block. This block is used by RTI to store internal model dependent data. Deleting this block will result in data loss.
      |
      | NEVER DELETE, COPY, OR MODIFY THIS BLOCK!
      mask Help:
      | RTI Data Store Block. This block is used by RTI to store internal model dependent data. Deleting this block will result in data loss.
      | 
      | NEVER DELETE, COPY, OR MODIFY THIS BLOCK!
      mask Display: text(0.5, 0.5, ' ', 'HorizontalAlignment', 'center');

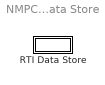
== system NMPC_4VEH_4TL/RTI Data/RTI Data Store/RTI Data Store ==
  RTI Data Store : Subsystem  mask(RTI_DATA_STORE){}
      mask help:
      | RTI Data Store Block. This block is used by RTI to store internal model dependent data. Deleting this block will result in data loss.
      |
      | NEVER DELETE, COPY, OR MODIFY THIS BLOCK!
      mask Help:
      | RTI Data Store Block. This block is used by RTI to store internal model dependent data. Deleting this block will result in data loss.
      | 
      | NEVER DELETE, COPY, OR MODIFY THIS BLOCK!
      mask Display: text(0.5, 0.5, ' ', 'HorizontalAlignment', 'center');

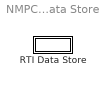
== system NMPC_4VEH_4TL/RTI Data/RTI Data Store/RTI Data Store/RTI Data Store ==
  RTI Data Store : Subsystem  mask(RTI_DATA_STORE){}
      mask help:
      | RTI Data Store Block. This block is used by RTI to store internal model dependent data. Deleting this block will result in data loss.
      |
      | NEVER DELETE, COPY, OR MODIFY THIS BLOCK!
      mask Help:
      | RTI Data Store Block. This block is used by RTI to store internal model dependent data. Deleting this block will result in data loss.
      | 
      | NEVER DELETE, COPY, OR MODIFY THIS BLOCK!
      mask Display: text(0.5, 0.5, ' ', 'HorizontalAlignment', 'center');

== system NMPC_4VEH_4TL/RTI Data/RTI Data Store/RTI Data Store/RTI Data Store/RTI Data Store ==

== matlab function NMPC_4VEH_4TL/NMPC WITH MOTOR DYNAMICS/flag_Stop ==
  data: state input; time input; online_data input; flag_old input; time_flag_memory input; flag_mpc output size=[1,7]; time_flag output size=[1 7]; t_dwell input
function [flag_mpc, time_flag] = fcn(state, time, online_data, flag_old, time_flag_memory, t_dwell)

s_stop = [80, 447, 756, 1084, 1304, 1507, 1822];
N_stop = length(s_stop);

flag_mpc = zeros(1,N_stop);
time_flag = time_flag_memory(:).';

for jj = 1:N_stop

    if state(2) < 0.01 && abs(s_stop(jj) - state(1)) < 0.5

        if time_flag_memory(jj) == 0
            time_flag(1,jj) = time;
            flag_mpc(1,jj) = 1;
        else
            if time - time_flag_memory(jj) > t_dwell
                flag_mpc(1,jj) = 0;
            else
                flag_mpc(1,jj) = 1;
            end
        end

    else
        flag_mpc(1,jj) = 0;
    end

end

== matlab function NMPC_4VEH_4TL/NMPC WITH MOTOR DYNAMICS/PLANT integration ==
  data: u input; s output; s0 input; v0 input; a0 input; red_stopline_hold input; s_hold input; u2 input; s02 input; v02 input; a02 input; red_stopline_hold2 input; s_hold2 input; u3 input; s03 input; v03 input; a03 input; red_stopline_hold3 input; s_hold3 input; u4 input; s04 input; v04 input; a04 input; red_stopline_hold4 input; s_hold4 input; v output; a output; s2 output; v2 output; a2 output; s3 output; v3 output; a3 output; s4 output; v4 output; a4 output; stop_flag output
function [s, v, a, s2, v2, a2, s3, v3, a3, s4, v4, a4, stop_flag] = plant_integrator( ...
    u,  s0,  v0,  a0,  red_stopline_hold,  s_hold, ...
    u2, s02, v02, a02, red_stopline_hold2, s_hold2, ...
    u3, s03, v03, a03, red_stopline_hold3, s_hold3, ...
    u4, s04, v04, a04, red_stopline_hold4, s_hold4)

%==========================================================================
% PLANT INTEGRATOR - 4 VEHICLES
%==========================================================================

dt = 0.1;
Ax_min = -1.5;
Ax_max =  1.5;

% Fine percorso: i veicoli vengono congelati quando raggiungono queste posizioni.
% La simulazione termina quando tutti e 4 le hanno raggiunte.
s_path_end1 = 5150;   % [m] veh1 - fine percorso 30TL
s_path_end2 = 5120;   % [m] veh2 - fine percorso 30TL
s_path_end3 = 5090;   % [m] veh3 - fine percorso 30TL
s_path_end4 = 5060;   % [m] veh4 - fine percorso 30TL

path_end_hold1 = (s0  >= s_path_end1);
path_end_hold2 = (s02 >= s_path_end2);
path_end_hold3 = (s03 >= s_path_end3);
path_end_hold4 = (s04 >= s_path_end4);

%==========================================================================
% VEHICLE 1
%==========================================================================

if red_stopline_hold
    s = min(s0, s_hold);
    v = 0;
    a = 0;
elseif path_end_hold1
    s = s_path_end1;
    v = 0;
    a = 0;
else
    a = a0 + u*dt;
    if a > Ax_max
        a = Ax_max;
    elseif a < Ax_min
        a = Ax_min;
    end
    v = v0 + a*dt;
    if v < 0
        v = 0;
    end
    s = s0 + v*dt;
end

%==========================================================================
% VEHICLE 2
%==========================================================================

if red_stopline_hold2
    s2 = min(s02, s_hold2);
    v2 = 0;
    a2 = 0;
elseif path_end_hold2
    s2 = s_path_end2;
    v2 = 0;
    a2 = 0;
else
    a2 = a02 + u2*dt;
    if a2 > Ax_max
        a2 = Ax_max;
    elseif a2 < Ax_min
        a2 = Ax_min;
    end
    v2 = v02 + a2*dt;
    if v2 < 0
        v2 = 0;
    end
    s2 = s02 + v2*dt;
end

%==========================================================================
% VEHICLE 3
%==========================================================================

if red_stopline_hold3
    s3 = min(s03, s_hold3);
    v3 = 0;
    a3 = 0;
elseif path_end_hold3
    s3 = s_path_end3;
    v3 = 0;
    a3 = 0;
else
    a3 = a03 + u3*dt;
    if a3 > Ax_max
        a3 = Ax_max;
    elseif a3 < Ax_min
        a3 = Ax_min;
    end
    v3 = v03 + a3*dt;
    if v3 < 0
        v3 = 0;
    end
    s3 = s03 + v3*dt;
end

%==========================================================================
% VEHICLE 4
%==========================================================================

if red_stopline_hold4
    s4 = min(s04, s_hold4);
    v4 = 0;
    a4 = 0;
elseif path_end_hold4
    s4 = s_path_end4;
    v4 = 0;
    a4 = 0;
else
    a4 = a04 + u4*dt;
    if a4 > Ax_max
        a4 = Ax_max;
    elseif a4 < Ax_min
        a4 = Ax_min;
    end
    v4 = v04 + a4*dt;
    if v4 < 0
        v4 = 0;
    end
    s4 = s04 + v4*dt;
end

% Stop flag: tutti e 4 a fine percorso
stop_flag = path_end_hold1 && path_end_hold2 && path_end_hold3 && path_end_hold4;

end

== matlab function NMPC_4VEH_4TL/NMPC WITH MOTOR DYNAMICS/flag_Traffic_Light ==
  data: state input; jerk input; x_TL input; x_TL_old input; online_data input; flag_old input; flag_mpc output
function flag_mpc = fcn(state, jerk, x_TL, x_TL_old, online_data, flag_old)

s_TL = [45.5, 203.2, 384.2, 589.4, 773.6, 1004.2, 1225.3, 1419.7, 1507.8, 1739.0, ...
        1823.0, 1948.9, 2046.6, 2287.9, 2421.5, 2635.8, 2683.8, 2773.9, 2800.2, 2828.4, ...
        2981.4, 3232.6, 3420.6, 3600.4, 3764.9, 4051.8, 4215.6, 4434.6, 4648.9, 5107.8];

s_max = 5200;
N = 50;
N_od = 50;
N_TL = 30;

flag_mpc = zeros(1,N_TL);
flag_old = flag_old(:).';

for ii = 1:N_TL

    x_now = x_TL(1,ii);
    x_old = x_TL_old(1,ii);

    if x_now == x_old
        flag_old(1,ii) = flag_old(1,ii);
    else
        flag_old(1,ii) = 0;
    end

    if x_now == 0
        if state(2) < 0.1 && abs(s_TL(ii) - state(1)) < 0.5
            flag_mpc(1,ii) = 1;
        else
            flag_mpc(1,ii) = 0;
        end
    else
        if abs(s_max - state(1)) < 0.5 && flag_old(1,ii) == 1
            flag_mpc(1,ii) = 1;
        else
            flag_mpc(1,ii) = 0;
        end
    end

    if state(1) >= s_TL(ii) || sum(online_data(ii:N_od:end)) == N+1
        flag_mpc(1,ii) = 0;
    end

end

== matlab function NMPC_4VEH_4TL/NMPC WITH MOTOR DYNAMICS/Traffic Light planner ==
  data: time_bag input; x_TL output size=[36 30]; tl_col input; time input; data output size=[36 30]; t_offset input; time_grid input
function [x_TL,data] = get_TL_data( ...
    time_bag, tl_col, time, t_offset, time_grid)
%#codegen
%==========================================================================
% TRAFFIC LIGHT PREVIEW SU GRIGLIA NMPC NON UNIFORME
%==========================================================================
% Costruisce il preview semaforico sui 45 nodi della griglia Chebyshev.
%
% Convenzione:
%   x_TL = 1 -> verde / vincolo rilasciato
%   x_TL = 0 -> rosso / vincolo attivo
%
% INPUT:
%   time_bag : vettore temporale associato alle righe di tl_col
%   tl_col   : matrice dei colori semaforici
%   time     : tempo corrente della simulazione
%   t_offset : offset applicato al preview usato dal NMPC
%   time_grid: nodi temporali NMPC, dimensione 45x1
%
% OUTPUT:
%   x_TL : preview con offset, dimensione 45 x N_tl
%   data : preview senza offset, usato per diagnostica
%==========================================================================

N = 35;
N_nodes = N + 1;

n_tl   = size(tl_col,2);
n_rows = size(tl_col,1);

x_TL = zeros(N_nodes,n_tl);
data = zeros(N_nodes,n_tl);

%--------------------------------------------------------------------------
% Passo temporale dei dati semaforici
%--------------------------------------------------------------------------
% Questa forma funziona sia con:
%   time_bag = 0:0.1:...
% sia con:
%   time_bag = 0:1:...
% purché time_bag e tl_col siano coerenti.

if length(time_bag) >= 2

    Ts_spat = time_bag(2)-time_bag(1);

else

    Ts_spat = 1.0;

end

% Protezione da dati temporali non validi
if ~isfinite(Ts_spat) || Ts_spat <= 0
    Ts_spat = 1.0;
end

if length(time_bag) >= 1

    t_data_start = time_bag(1);

else

    t_data_start = 0.0;

end

%==========================================================================
% PREVIEW SEMAFORICO CON OFFSET
%==========================================================================
% Questo è il preview utilizzato dal controllore NMPC.

for kk = 1:N_nodes

    % Tempo assoluto corrispondente al nodo Chebyshev kk
    t_k = time + t_offset + time_grid(kk);

    % Zero-order hold:
    % viene selezionato l'ultimo valore disponibile prima di t_k
    eta = (t_k-t_data_start)/Ts_spat;

    row = floor(eta)+1;

    % Saturazione agli estremi della tabella
    row = max(1,min(row,n_rows));

    x_TL(kk,:) = tl_col(row,:);

end

%==========================================================================
% PREVIEW SEMAFORICO SENZA OFFSET
%==========================================================================
% Usato soltanto per diagnostica e confronto con il segnale reale.

for kk = 1:N_nodes

    t_k = time + time_grid(kk);

    eta = (t_k-t_data_start)/Ts_spat;

    row = floor(eta)+1;

    row = max(1,min(row,n_rows));

    data(kk,:) = tl_col(row,:);

end

end

== matlab function NMPC_4VEH_4TL/NMPC WITH MOTOR DYNAMICS/MATLAB Function ==
  data: flag output; state_pred input; NMPC_Wmat1 output
function [flag, NMPC_Wmat1] = fcn(state_pred)

% pos_hor = state_pred(:,1);
% if pos_hor(1) > 1500 && pos_hor(1) < 1800
%     flag = 0;
% else
%     flag = 1;
% end
flag=0;

 Qx1 = [30 20 10 2 2 2 0.5 0.5 0.5 50 50 50 200 200 200 500 500 500 100 100 100 0.1 0.1];
 W1 = diag(Qx1);
 NMPC_Wmat1 = reshape(W1.',1,[]);

== matlab function NMPC_4VEH_4TL/NMPC WITH MOTOR DYNAMICS/ROAD PREVIEW/road_curvature_preview ==
  data: pos_hor input; k_road_hor output; s_start input; ds_map input; k_road_map input
function k_road_hor = RoadCurvaturePreview( ...
    pos_hor, s_start, ds_map, k_road_map)
%#codegen
%==========================================================================
% ROAD CURVATURE PREVIEW
%==========================================================================
% Calcola la curvatura stradale nei 45 nodi predittivi del NMPC.
%
% La griglia temporale non compare esplicitamente perché pos_hor contiene
% già le posizioni predette nei nodi della griglia Chebyshev:
%
%   pos_hor(1)  -> t = time_grid(1)
%   pos_hor(2)  -> t = time_grid(2)
%   ...
%   pos_hor(45) -> t = time_grid(45)
%
% INPUT:
%   pos_hor   : posizione predetta, dimensione 45x1
%   s_start   : coordinata iniziale della mappa
%   ds_map    : passo spaziale della lookup table
%   k_road_map: valori della curvatura
%
% OUTPUT:
%   k_road_hor: curvatura nei 45 nodi, dimensione 45x1
%==========================================================================

N = 35;
N_nodes = N + 1;

k_road_hor = zeros(N_nodes,1);

n_map = length(k_road_map);

for kk = 1:N_nodes

    % Posizione predetta al nodo kk
    s_pred = pos_hor(kk);

    % Indice continuo nella lookup table
    eta = (s_pred - s_start)/ds_map + 1;

    % Indice inferiore e coefficiente di interpolazione
    idx0  = floor(eta);
    alpha = eta - idx0;

    % Saturazione agli estremi della mappa
    if idx0 < 1

        k_val = k_road_map(1);

    elseif idx0 >= n_map

        k_val = k_road_map(n_map);

    else

        % Interpolazione lineare spaziale
        k0 = k_road_map(idx0);
        k1 = k_road_map(idx0 + 1);

        k_val = k0 + alpha*(k1-k0);

    end

    % Protezione numerica
    if ~isfinite(k_val)
        k_val = 0;
    end

    % Il vincolo laterale usa il valore assoluto della curvatura
    k_road_hor(kk) = abs(k_val);

end

end

== matlab function NMPC_4VEH_4TL/NMPC WITH MOTOR DYNAMICS/ROAD PREVIEW/road_curvature_preview1 ==
  data: pos_hor_2 input; k_road_hor_2 output; s_start_2 input; ds_map input; k_road_map input
function k_road_hor_2 = RoadCurvaturePreview( ...
    pos_hor_2, s_start_2, ds_map, k_road_map)
%#codegen
%==========================================================================
% ROAD CURVATURE PREVIEW
%==========================================================================
% Calcola la curvatura stradale nei 45 nodi predittivi del NMPC.
%
% La griglia temporale non compare esplicitamente perché pos_hor_2 contiene
% già le posizioni predette nei nodi della griglia Chebyshev:
%
%   pos_hor_2(1)  -> t = time_grid(1)
%   pos_hor_2(2)  -> t = time_grid(2)
%   ...
%   pos_hor_2(45) -> t = time_grid(45)
%
% INPUT:
%   pos_hor_2   : posizione predetta, dimensione 45x1
%   s_start_2   : coordinata iniziale della mappa
%   ds_map    : passo spaziale della lookup table
%   k_road_map: valori della curvatura
%
% OUTPUT:
%   k_road_hor_2: curvatura nei 45 nodi, dimensione 45x1
%==========================================================================

N = 35;
N_nodes = N + 1;

k_road_hor_2 = zeros(N_nodes,1);

n_map = length(k_road_map);

for kk = 1:N_nodes

    % Posizione predetta al nodo kk
    s_pred = pos_hor_2(kk);

    % Indice continuo nella lookup table
    eta = (s_pred - s_start_2)/ds_map + 1;

    % Indice inferiore e coefficiente di interpolazione
    idx0  = floor(eta);
    alpha = eta - idx0;

    % Saturazione agli estremi della mappa
    if idx0 < 1

        k_val = k_road_map(1);

    elseif idx0 >= n_map

        k_val = k_road_map(n_map);

    else

        % Interpolazione lineare spaziale
        k0 = k_road_map(idx0);
        k1 = k_road_map(idx0 + 1);

        k_val = k0 + alpha*(k1-k0);

    end

    % Protezione numerica
    if ~isfinite(k_val)
        k_val = 0;
    end

    % Il vincolo laterale usa il valore assoluto della curvatura
    k_road_hor_2(kk) = abs(k_val);

end

end

== matlab function NMPC_4VEH_4TL/NMPC WITH MOTOR DYNAMICS/TIC ==
  data: y output; u input
function y = fcn(u)
% The output y is of size 2x1.
%
% Zihao Liu 23/5/2020
% Last Change 23/5/2020

y = zeros(2,1);
t = tic; % During Code Gen, MATLAB returns a struct contains tv_sec and tv_nsec.
y(1) = t.tv_sec;
y(2) = t.tv_nsec;


end

== matlab function NMPC_4VEH_4TL/NMPC WITH MOTOR DYNAMICS/TOC ==
  data: u input; y output
function y = fcn(u)
% Output y is a double scaler, in seconds.
%
%
% Zihao Liu 23/5/2020
% Last Change 23/5/2020


% Reconstruct the struct from tic.
t.tv_sec = u(1);
t.tv_nsec = u(2);
y = toc(t);

end

== matlab function NMPC_4VEH_4TL/NMPC WITH MOTOR DYNAMICS/ROAD PREVIEW/road_curvature_preview2 ==
  data: pos_hor_3 input; k_road_hor_3 output; s_start_3 input; ds_map input; k_road_map input
function k_road_hor_3 = RoadCurvaturePreview( ...
    pos_hor_3, s_start_3, ds_map, k_road_map)
%#codegen
%==========================================================================
% ROAD CURVATURE PREVIEW
%==========================================================================
% Calcola la curvatura stradale nei 45 nodi predittivi del NMPC.
%
% La griglia temporale non compare esplicitamente perché pos_hor_3 contiene
% già le posizioni predette nei nodi della griglia Chebyshev:
%
%   pos_hor_3(1)  -> t = time_grid(1)
%   pos_hor_3(2)  -> t = time_grid(2)
%   ...
%   pos_hor_3(45) -> t = time_grid(45)
%
% INPUT:
%   pos_hor_3   : posizione predetta, dimensione 45x1
%   s_start_3   : coordinata iniziale della mappa
%   ds_map    : passo spaziale della lookup table
%   k_road_map: valori della curvatura
%
% OUTPUT:
%   k_road_hor_3: curvatura nei 45 nodi, dimensione 45x1
%==========================================================================

N = 35;
N_nodes = N + 1;

k_road_hor_3 = zeros(N_nodes,1);

n_map = length(k_road_map);

for kk = 1:N_nodes

    % Posizione predetta al nodo kk
    s_pred = pos_hor_3(kk);

    % Indice continuo nella lookup table
    eta = (s_pred - s_start_3)/ds_map + 1;

    % Indice inferiore e coefficiente di interpolazione
    idx0  = floor(eta);
    alpha = eta - idx0;

    % Saturazione agli estremi della mappa
    if idx0 < 1

        k_val = k_road_map(1);

    elseif idx0 >= n_map

        k_val = k_road_map(n_map);

    else

        % Interpolazione lineare spaziale
        k0 = k_road_map(idx0);
        k1 = k_road_map(idx0 + 1);

        k_val = k0 + alpha*(k1-k0);

    end

    % Protezione numerica
    if ~isfinite(k_val)
        k_val = 0;
    end

    % Il vincolo laterale usa il valore assoluto della curvatura
    k_road_hor_3(kk) = abs(k_val);

end

end
